simulink model "Controller_without_ref"  (R2015b)
settings: Solver=FixedStepDiscrete  SolverMode=SingleTasking  StartTime=0.0  StopTime=inf  RelTol=1e-3
undefined symbols (not defined in the file or in its folder): Controls, DiscIntNeverNeededParam, GroupMix
libraries: robotlib x34, simulink x6
settings Model: Creator=rasrack  LastModifiedBy=rasrack
settings OptimizationCC: DefaultParameterBehavior=Inlined  UseFloatMulNetSlope=on  InlineInvariantSignals=on  PassReuseOutputArgsAs=Individual arguments  ZeroExternalMemoryAtStartup=off  ZeroInternalMemoryAtStartup=off  NoFixptDivByZeroProtection=on  EfficientFloat2IntCast=on  OptimizeModelRefInitCode=on  LifeSpan=1  MaxStackSize=64
settings HardwareCC: ProdBitPerPointer=32  ProdLargestAtomicFloat=None  ProdIntDivRoundTo=Undefined  ProdEndianess=Unspecified  ProdWordSize=32  ProdHWDeviceType=Generic->Unspecified (assume 32-bit Generic)
settings ModelReferenceCC: EnableParallelModelReferenceBuilds=on
settings RTWCC: SystemTargetFile=ert.tlc  GenCodeOnly=on  TemplateMakefile=ert_default_tmf  Description=Embedded Coder  GenerateReport=on  Toolchain=Catkin  IncludeHyperlinkInReport=on  LaunchReport=on  TargetLang=C++  GenerateTraceInfo=on  GenerateTraceReport=on  GenerateTraceReportSl=on  GenerateTraceReportSf=on  GenerateTraceReportEml=on
settings CodeAppCC: ForceParamTrailComments=on  IgnoreCustomStorageClasses=off  SimulinkDataObjDesc=on  InsertBlockDesc=on  InternalIdentifier=Classic  ReqsInCode=on
settings ERTTargetCC: IncludeMdlTerminateFcn=off  CombineSignalStateStructs=on  MultiInstanceERTCode=on  CodeInterfacePackaging=C++ class  SupportNonFinite=off  SupportVariableSizeSignals=on  InlinedParameterPlacement=NonHierarchical  RootIOFormat=Structure reference  ERTFilePackagingFormat=CompactWithDataFile

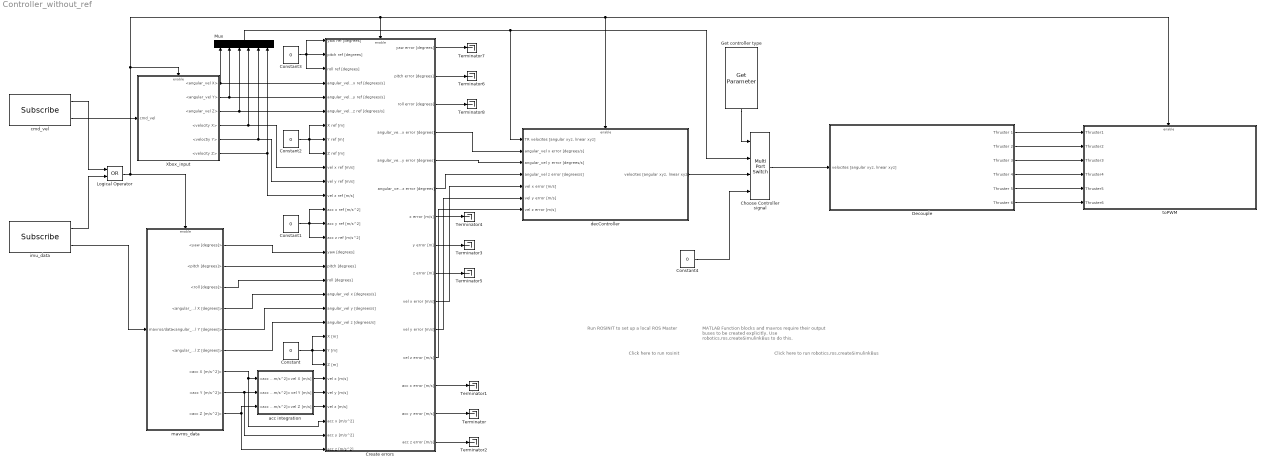
== system Controller_without_ref ==
  note: Click here to run
      | robotics.ros.createSimulinkBus
  note: Run ROSINIT to set up a local ROS Master
  note: MATLAB Function blocks and mavros require their output buses to be created explicitly. Use robotics.ros.createSimulinkBus to do this.
  note: Click here to run
      | rosinit
  Choose Controller signal : MultiPortSwitch  DataPortOrder=Specify indices  DataPortIndices={0,1,2}
  Constant{,1..4} (5 alike) : Constant  Value=0
  Create errors : Subsystem
  Decouple : Subsystem
  Get controller type : robotlib/Get Parameter  SourceLibraryInfo=This block requires Robotics System Toolbox  ParameterSource=Select from ROS network  ParameterName=/matlab_controller/controller  ParameterType=int32  ParameterInitialValue=0  SampleTime=-1  ShowErrorCodeOutput=off  ModelName=Controller_without_ref  BlockId=ParamGet_Controller_without_ref_106
  Logical Operator : Logic  Operator=OR  AllPortsSameDT=off  OutDataTypeStr=boolean
  Mux : Mux  Inputs=6
  Terminator{,1..8} (9 alike) : Terminator
  Xbox_input : Subsystem
  acc integration : Subsystem
  cmd_vel : robotlib/Subscribe  SourceLibraryInfo=This block requires Robotics System Toolbox  topicSource=Select from ROS network  topic=/cmd_vel  messageType=geometry_msgs/Twist  sampleTime=-1  messageQueueLength=10
  decController : Subsystem
  imu_data : robotlib/Subscribe  SourceLibraryInfo=This block requires Robotics System Toolbox  topicSource=Select from ROS network  topic=/mavros/imu/data  messageType=sensor_msgs/Imu  sampleTime=-1  messageQueueLength=10
  mavros_data : Subsystem  TreatAsAtomicUnit=on
  toPWM : Subsystem
  wires:
  cmd_vel/2 -> Xbox_input/1(cmd_vel)
  cmd_vel/1 -> Logical Operator/1
  imu_data/1 -> Logical Operator/2
  imu_data/2 -> mavros_data/1(mavros/data)
  Get controller type/1 -> Choose Controller signal/1
  Xbox_input/1(<angular_vel X>) -> Create errors/4(angular_vel x ref [degrees/s]), Mux/1
  Xbox_input/2(<angular_vel Y>) -> Mux/2, Create errors/5(angular_vel y ref [degrees/s])
  Xbox_input/3("<angular_vel Z> ") -> Mux/3, Create errors/6("angular_vel z ref [degrees/s] ")
  Xbox_input/4(<velocity X>) -> Mux/4, Create errors/10(vel x ref [m/s])
  Xbox_input/5(<veloctiy Y>) -> Mux/5, Create errors/11(vel y ref [m/s])
  Xbox_input/6(<velocity Z>) -> Create errors/12(vel z ref [m/s]), Mux/6
  mavros_data/1(<yaw [degrees]>) -> Create errors/16("yaw [degrees]  ")
  mavros_data/2(<pitch [degrees]>) -> Create errors/17(pitch [degrees])
  mavros_data/3(<roll [degrees]>) -> Create errors/18(roll [degrees])
  mavros_data/4(<angular_vel X [degrees]>) -> Create errors/19("angular_vel x [degrees/s]  ")
  mavros_data/5(<angular_vel Y [degrees]>) -> Create errors/20("angular_vel y [degrees/s] ")
  mavros_data/6(<angular_vel Z [degrees]>) -> Create errors/21(angular_vel z [degrees/s])
  Constant/1 -> Create errors/22(X [m]), Create errors/24(Z [m]), Create errors/23(Y [m])
  acc integration/2(vel Y [m/s]) -> Create errors/26(vel y [m/s])
  acc integration/1("vel X [m/s] ") -> Create errors/25(vel x [m/s])
  acc integration/3(vel Z [m/s]) -> Create errors/27(vel z [m/s])
  mavros_data/7(<acc X [m/s^2]>) -> Create errors/28(acc x [m/s^2]), acc integration/1("<acc X [m/s^2]> ")
  mavros_data/8(<acc Y [m/s^2]>) -> Create errors/29(acc y [m/s^2]), acc integration/2(<acc Y [m/s^2]>)
  mavros_data/9(<acc Z [m/s^2]>) -> Create errors/30(acc z [m/s^2]), acc integration/3(<acc Z [m/s^2]>)
  Constant1/1 -> Create errors/15(acc z ref [m/s^2]), Create errors/13(acc x ref [m/s^2]), Create errors/14(acc y ref [m/s^2])
  Constant2/1 -> Create errors/9(Z ref [m]), Create errors/7(X ref [m]), Create errors/8(Y ref [m])
  Constant3/1 -> Create errors/1("yaw ref [degrees] "), Create errors/3(roll ref [degrees]), Create errors/2("pitch ref [degrees] ")
  Mux/1 -> decController/1("TR velocites [angular xyz, linear xyz]  "), Choose Controller signal/2
  Create errors/14(acc y error [m/s]) -> Terminator/1
  Create errors/13(acc x error [m/s]) -> Terminator1/1
  Create errors/15(acc z error [m/s]) -> Terminator2/1
  Create errors/8(y error [m]) -> Terminator3/1
  Create errors/7(x error [m/s]) -> Terminator4/1
  Create errors/9(z error [m]) -> Terminator5/1
  Create errors/2(pitch error [degrees]) -> Terminator6/1
  Create errors/1(yaw error [degrees]) -> Terminator7/1
  Create errors/3(roll error [degrees]) -> Terminator8/1
  Constant4/1 -> Choose Controller signal/4
  Choose Controller signal/1 -> Decouple/1("velocites [angular xyz, linear xyz]    ")
  Create errors/4(angular_vel x error [degrees]) -> decController/2("angular_vel x error [degrees/s] ")
  Create errors/5(angular_vel y error [degrees]) -> decController/3(angular_vel y error [degrees/s])
  Create errors/6(angular_vel z error [degrees]) -> decController/4(angular_vel z error [degrees/s])
  Create errors/10(vel x error [m/s]) -> decController/5("vel x error [m/s] ")
  Create errors/11(vel y error [m/s]) -> decController/6("vel y error [m/s] ")
  Create errors/12(vel z error [m/s]) -> decController/7("vel z error [m/s] ")
  decController/1("velocites [angular xyz, linear xyz]") -> Choose Controller signal/3
  Logical Operator/1 -> mavros_data/Enable, Create errors/Enable, toPWM/Enable, decController/Enable, Xbox_input/Enable
  Decouple/3(Thruster 3) -> toPWM/3(Thruster3)
  Decouple/2(Thruster 2) -> toPWM/2(Thruster2)
  Decouple/5(Thruster 5) -> toPWM/5(Thruster5)
  Decouple/1(Thruster 1) -> toPWM/1(Thruster1)
  Decouple/4(Thruster 4) -> toPWM/4(Thruster4)
  Decouple/6(Thruster 6) -> toPWM/6(Thruster6)

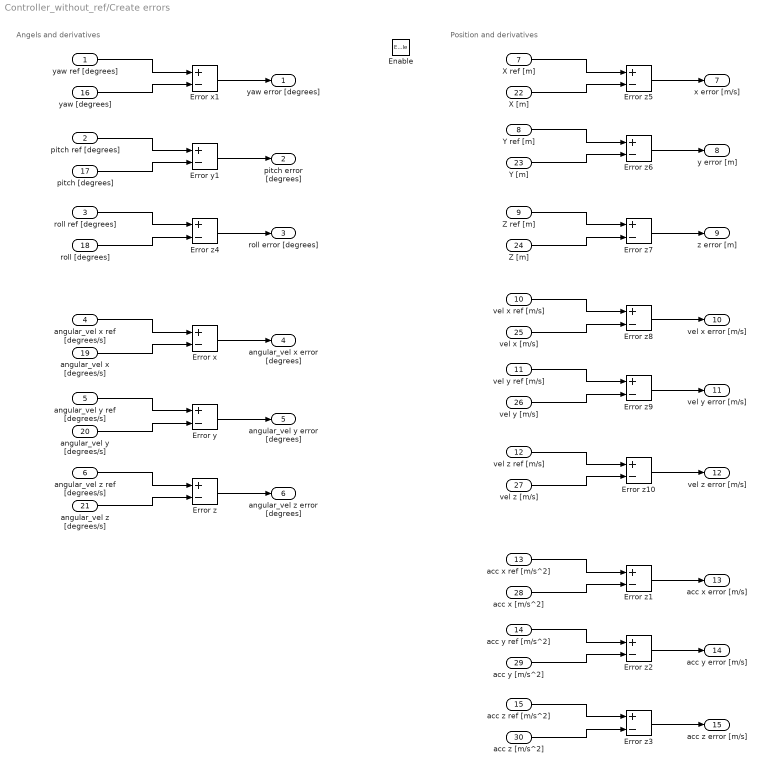
== system Controller_without_ref/Create errors ==
  note: Position and derivatives
  note: Angels and derivatives
  "yaw ref [degrees] " : Inport
  "pitch ref [degrees] " : Inport  Port=2
  roll ref [degrees] : Inport  Port=3
  angular_vel x ref [degrees/s] : Inport  Port=4
  angular_vel y ref [degrees/s] : Inport  Port=5
  "angular_vel z ref [degrees/s] " : Inport  Port=6
  X ref [m] : Inport  Port=7
  Y ref [m] : Inport  Port=8
  Z ref [m] : Inport  Port=9
  vel x ref [m/s] : Inport  Port=10
  vel y ref [m/s] : Inport  Port=11
  vel z ref [m/s] : Inport  Port=12
  acc x ref [m/s^2] : Inport  Port=13
  acc y ref [m/s^2] : Inport  Port=14
  acc z ref [m/s^2] : Inport  Port=15
  "yaw [degrees]  " : Inport  Port=16
  pitch [degrees] : Inport  Port=17
  roll [degrees] : Inport  Port=18
  "angular_vel x [degrees/s]  " : Inport  Port=19
  "angular_vel y [degrees/s] " : Inport  Port=20
  angular_vel z [degrees/s] : Inport  Port=21
  X [m] : Inport  Port=22
  Y [m] : Inport  Port=23
  Z [m] : Inport  Port=24
  vel x [m/s] : Inport  Port=25
  vel y [m/s] : Inport  Port=26
  vel z [m/s] : Inport  Port=27
  acc x [m/s^2] : Inport  Port=28
  acc y [m/s^2] : Inport  Port=29
  acc z [m/s^2] : Inport  Port=30
  Enable : EnablePort
  Error x : Sum  Inputs=+-
  Error x1 : Sum  Inputs=+-
  Error y : Sum  Inputs=+-
  Error y1 : Sum  Inputs=+-
  Error z{,1..10} (11 alike) : Sum  Inputs=+-
  yaw error [degrees] : Outport
  pitch error [degrees] : Outport  Port=2
  roll error [degrees] : Outport  Port=3
  angular_vel x error [degrees] : Outport  Port=4
  angular_vel y error [degrees] : Outport  Port=5
  angular_vel z error [degrees] : Outport  Port=6
  x error [m/s] : Outport  Port=7
  y error [m] : Outport  Port=8
  z error [m] : Outport  Port=9
  vel x error [m/s] : Outport  Port=10
  vel y error [m/s] : Outport  Port=11
  vel z error [m/s] : Outport  Port=12
  acc x error [m/s] : Outport  Port=13
  acc y error [m/s] : Outport  Port=14
  acc z error [m/s] : Outport  Port=15
  wires:
  angular_vel x ref [degrees/s]/1 -> Error x/1
  "angular_vel x [degrees/s]  "/1 -> Error x/2
  Error x/1 -> angular_vel x error [degrees]/1
  angular_vel y ref [degrees/s]/1 -> Error y/1
  "angular_vel y [degrees/s] "/1 -> Error y/2
  Error y/1 -> angular_vel y error [degrees]/1
  "angular_vel z ref [degrees/s] "/1 -> Error z/1
  angular_vel z [degrees/s]/1 -> Error z/2
  Error z/1 -> angular_vel z error [degrees]/1
  acc x ref [m/s^2]/1 -> Error z1/1
  acc x [m/s^2]/1 -> Error z1/2
  Error z1/1 -> acc x error [m/s]/1
  acc y ref [m/s^2]/1 -> Error z2/1
  acc y [m/s^2]/1 -> Error z2/2
  Error z2/1 -> acc y error [m/s]/1
  acc z ref [m/s^2]/1 -> Error z3/1
  acc z [m/s^2]/1 -> Error z3/2
  Error z3/1 -> acc z error [m/s]/1
  "yaw ref [degrees] "/1 -> Error x1/1
  "yaw [degrees]  "/1 -> Error x1/2
  Error x1/1 -> yaw error [degrees]/1
  "pitch ref [degrees] "/1 -> Error y1/1
  pitch [degrees]/1 -> Error y1/2
  Error y1/1 -> pitch error [degrees]/1
  roll ref [degrees]/1 -> Error z4/1
  roll [degrees]/1 -> Error z4/2
  Error z4/1 -> roll error [degrees]/1
  X ref [m]/1 -> Error z5/1
  X [m]/1 -> Error z5/2
  Error z5/1 -> x error [m/s]/1
  Y ref [m]/1 -> Error z6/1
  Y [m]/1 -> Error z6/2
  Error z6/1 -> y error [m]/1
  Z ref [m]/1 -> Error z7/1
  Z [m]/1 -> Error z7/2
  Error z7/1 -> z error [m]/1
  vel x ref [m/s]/1 -> Error z8/1
  vel x [m/s]/1 -> Error z8/2
  Error z8/1 -> vel x error [m/s]/1
  vel y ref [m/s]/1 -> Error z9/1
  vel y [m/s]/1 -> Error z9/2
  Error z9/1 -> vel y error [m/s]/1
  vel z ref [m/s]/1 -> Error z10/1
  vel z [m/s]/1 -> Error z10/2
  Error z10/1 -> vel z error [m/s]/1

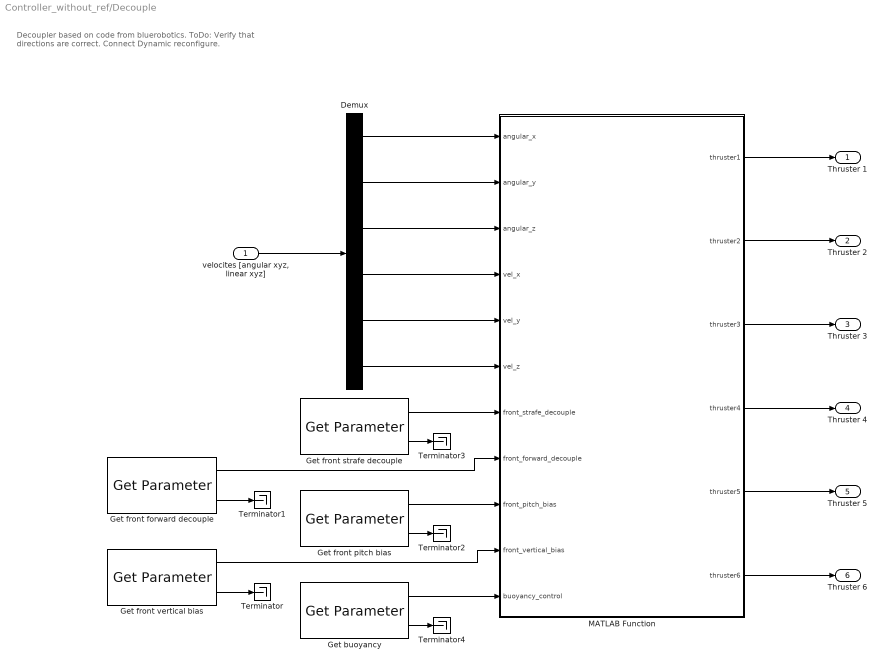
== system Controller_without_ref/Decouple ==
  note: Decoupler based on code from bluerobotics.
      | ToDo:
      | Verify that directions are correct.
      | Connect Dynamic reconfigure.
  "velocites [angular xyz, linear xyz]    " : Inport
  Demux : Demux  Outputs=6
  Get buoyancy : robotlib/Get Parameter  SourceLibraryInfo=This block requires Robotics System Toolbox  ParameterSource=Select from ROS network  ParameterName=/matlab_controller/buoyancy_control  ParameterType=double  ParameterInitialValue=0.0  SampleTime=-1  ShowErrorCodeOutput=on  ModelName=Controller_without_ref  BlockId=ParamGet_Controller_without_ref_462
  Get front forward decouple : robotlib/Get Parameter  SourceLibraryInfo=This block requires Robotics System Toolbox  ParameterSource=Select from ROS network  ParameterName=/matlab_controller/front_forward_decouple  ParameterType=double  ParameterInitialValue=0.0  SampleTime=-1  ShowErrorCodeOutput=on  ModelName=Controller_without_ref  BlockId=ParamGet_Controller_without_ref_463
  Get front pitch bias : robotlib/Get Parameter  SourceLibraryInfo=This block requires Robotics System Toolbox  ParameterSource=Select from ROS network  ParameterName=/matlab_controller/front_pitch_bias  ParameterType=double  ParameterInitialValue=0.0  SampleTime=-1  ShowErrorCodeOutput=on  ModelName=Controller_without_ref  BlockId=ParamGet_Controller_without_ref_464
  Get front strafe decouple : robotlib/Get Parameter  SourceLibraryInfo=This block requires Robotics System Toolbox  ParameterSource=Select from ROS network  ParameterName=/matlab_controller/front_strafe_decouple  ParameterType=double  ParameterInitialValue=0.0  SampleTime=-1  ShowErrorCodeOutput=on  ModelName=Controller_without_ref  BlockId=ParamGet_Controller_without_ref_465
  Get front vertical bias : robotlib/Get Parameter  SourceLibraryInfo=This block requires Robotics System Toolbox  ParameterSource=Select from ROS network  ParameterName=/matlab_controller/front_vertical_bias  ParameterType=double  ParameterInitialValue=0.0  SampleTime=-1  ShowErrorCodeOutput=on  ModelName=Controller_without_ref  BlockId=ParamGet_Controller_without_ref_466
  MATLAB Function : MATLAB Function  TreatAsAtomicUnit=on
  Terminator{,1..4} (5 alike) : Terminator
  Thruster 1 : Outport
  Thruster 2 : Outport  Port=2
  Thruster 3 : Outport  Port=3
  Thruster 4 : Outport  Port=4
  Thruster 5 : Outport  Port=5
  Thruster 6 : Outport  Port=6
  wires:
  MATLAB Function/1(thruster1) -> Thruster 1/1
  Get buoyancy/1 -> MATLAB Function/11(buoyancy_control)
  Get front vertical bias/1 -> MATLAB Function/10(front_vertical_bias)
  Get front pitch bias/1 -> MATLAB Function/9(front_pitch_bias)
  Get front forward decouple/1 -> MATLAB Function/8(front_forward_decouple)
  Get front strafe decouple/1 -> MATLAB Function/7(front_strafe_decouple)
  Demux/5 -> MATLAB Function/5(vel_y)
  Demux/6 -> MATLAB Function/6(vel_z)
  Demux/4 -> MATLAB Function/4(vel_x)
  Demux/3 -> MATLAB Function/3(angular_z)
  Demux/2 -> MATLAB Function/2(angular_y)
  Demux/1 -> MATLAB Function/1(angular_x)
  MATLAB Function/6(thruster6) -> Thruster 6/1
  MATLAB Function/5(thruster5) -> Thruster 5/1
  MATLAB Function/4(thruster4) -> Thruster 4/1
  MATLAB Function/3(thruster3) -> Thruster 3/1
  MATLAB Function/2(thruster2) -> Thruster 2/1
  Get front vertical bias/2 -> Terminator/1
  Get front forward decouple/2 -> Terminator1/1
  Get front pitch bias/2 -> Terminator2/1
  Get front strafe decouple/2 -> Terminator3/1
  Get buoyancy/2 -> Terminator4/1
  "velocites [angular xyz, linear xyz]    "/1 -> Demux/1

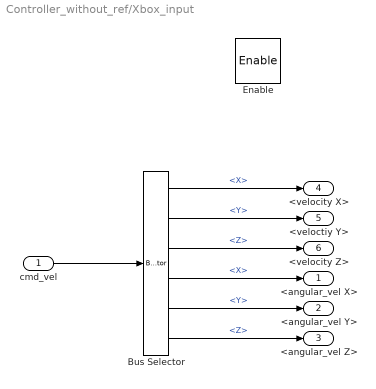
== system Controller_without_ref/Xbox_input ==
  cmd_vel : Inport
  Enable : EnablePort
  Bus Selector : BusSelector  OutputSignals=Linear.X,Linear.Y,Linear.Z,Angular.X,Angular.Y,Angular.Z
  <angular_vel X> : Outport
  <angular_vel Y> : Outport  Port=2
  "<angular_vel Z> " : Outport  Port=3
  <velocity X> : Outport  Port=4
  <veloctiy Y> : Outport  Port=5
  <velocity Z> : Outport  Port=6
  wires:
  cmd_vel/1 -> Bus Selector/1
  Bus Selector/2 -> <veloctiy Y>/1  "<Y>"
  Bus Selector/1 -> <velocity X>/1  "<X>"
  Bus Selector/5 -> <angular_vel Y>/1  "<Y>"
  Bus Selector/3 -> <velocity Z>/1  "<Z>"
  Bus Selector/6 -> "<angular_vel Z> "/1  "<Z>"
  Bus Selector/4 -> <angular_vel X>/1  "<X>"

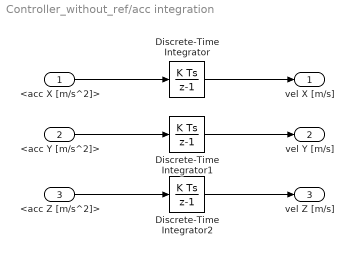
== system Controller_without_ref/acc integration ==
  "<acc X [m/s^2]> " : Inport
  <acc Y [m/s^2]> : Inport  Port=2
  <acc Z [m/s^2]> : Inport  Port=3
  Discrete-Time Integrator : DiscreteIntegrator  InitialConditionSetting=State (most efficient)  SampleTime=-1  ICPrevOutput=DiscIntNeverNeededParam  ICPrevScaledInput=DiscIntNeverNeededParam
  Discrete-Time Integrator1 : DiscreteIntegrator  InitialConditionSetting=State (most efficient)  SampleTime=-1  ICPrevOutput=DiscIntNeverNeededParam  ICPrevScaledInput=DiscIntNeverNeededParam
  Discrete-Time Integrator2 : DiscreteIntegrator  InitialConditionSetting=State (most efficient)  SampleTime=-1  ICPrevOutput=DiscIntNeverNeededParam  ICPrevScaledInput=DiscIntNeverNeededParam
  "vel X [m/s] " : Outport
  vel Y [m/s] : Outport  Port=2
  vel Z [m/s] : Outport  Port=3
  wires:
  "<acc X [m/s^2]> "/1 -> Discrete-Time Integrator/1
  <acc Y [m/s^2]>/1 -> Discrete-Time Integrator1/1
  <acc Z [m/s^2]>/1 -> Discrete-Time Integrator2/1
  Discrete-Time Integrator/1 -> "vel X [m/s] "/1
  Discrete-Time Integrator1/1 -> vel Y [m/s]/1
  Discrete-Time Integrator2/1 -> vel Z [m/s]/1

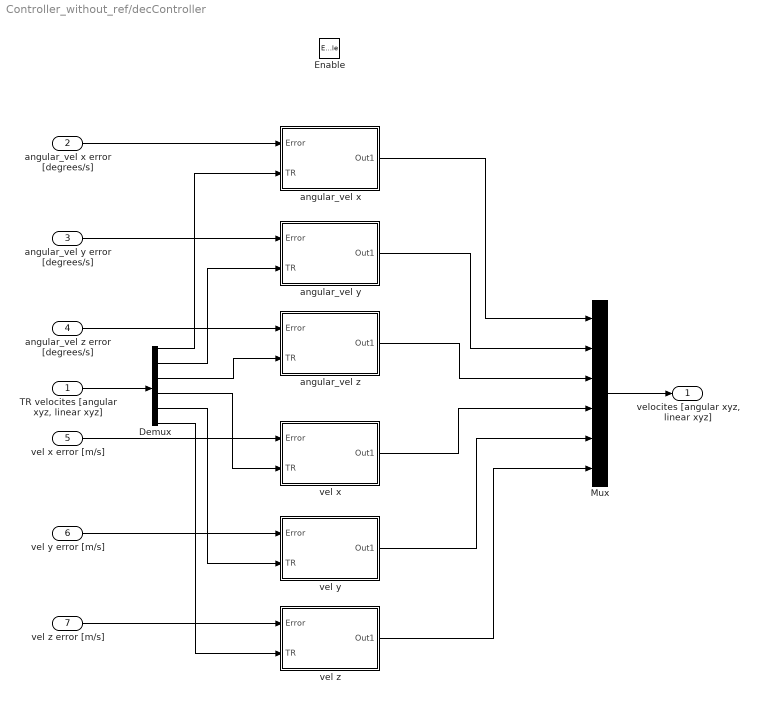
== system Controller_without_ref/decController ==
  "TR velocites [angular xyz, linear xyz]  " : Inport
  "angular_vel x error [degrees/s] " : Inport  Port=2
  angular_vel y error [degrees/s] : Inport  Port=3
  angular_vel z error [degrees/s] : Inport  Port=4
  "vel x error [m/s] " : Inport  Port=5
  "vel y error [m/s] " : Inport  Port=6
  "vel z error [m/s] " : Inport  Port=7
  Enable : EnablePort  OutDataTypeStr=boolean
  Demux : Demux  Outputs=6
  Mux : Mux  Inputs=6
  angular_vel x : Subsystem
  angular_vel y : Subsystem
  angular_vel z : Subsystem
  vel x : Subsystem
  vel y : Subsystem
  vel z : Subsystem
  "velocites [angular xyz, linear xyz]" : Outport
  wires:
  "angular_vel x error [degrees/s] "/1 -> angular_vel x/1(Error)
  angular_vel y error [degrees/s]/1 -> angular_vel y/1(Error)
  angular_vel z error [degrees/s]/1 -> angular_vel z/1(Error)
  "vel x error [m/s] "/1 -> vel x/1(Error)
  "vel y error [m/s] "/1 -> vel y/1(Error)
  "vel z error [m/s] "/1 -> vel z/1(Error)
  vel z/1(Out1) -> Mux/6
  angular_vel x/1(Out1) -> Mux/1
  angular_vel y/1(Out1) -> Mux/2
  angular_vel z/1(Out1) -> Mux/3
  vel x/1(Out1) -> Mux/4
  vel y/1(Out1) -> Mux/5
  Mux/1 -> "velocites [angular xyz, linear xyz]"/1
  "TR velocites [angular xyz, linear xyz]  "/1 -> Demux/1
  Demux/1 -> angular_vel x/2(TR)
  Demux/2 -> angular_vel y/2(TR)
  Demux/3 -> angular_vel z/2(TR)
  Demux/4 -> vel x/2(TR)
  Demux/5 -> vel y/2(TR)
  Demux/6 -> vel z/2(TR)

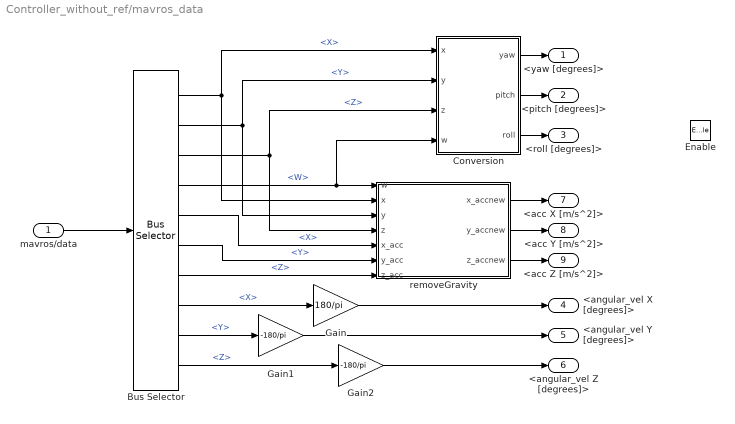
== system Controller_without_ref/mavros_data ==
  mavros/data : Inport
  Enable : EnablePort
  Bus Selector : BusSelector  OutputSignals=Orientation.X,Orientation.Y,Orientation.Z,Orientation.W,LinearAcceleration.X,LinearAcceleration.Y,LinearAcceleration.Z,AngularVelocity.X,AngularVelocity.Y,AngularVelocity.Z
  Conversion : MATLAB Function  TreatAsAtomicUnit=on
  Gain : Gain  Gain=180/pi
  Gain1 : Gain  Gain=-180/pi
  Gain2 : Gain  Gain=-180/pi
  removeGravity : MATLAB Function  TreatAsAtomicUnit=on
  <yaw [degrees]> : Outport
  <pitch [degrees]> : Outport  Port=2
  <roll [degrees]> : Outport  Port=3
  <angular_vel X [degrees]> : Outport  Port=4
  <angular_vel Y [degrees]> : Outport  Port=5
  <angular_vel Z [degrees]> : Outport  Port=6
  <acc X [m/s^2]> : Outport  Port=7
  <acc Y [m/s^2]> : Outport  Port=8
  <acc Z [m/s^2]> : Outport  Port=9
  wires:
  mavros/data/1 -> Bus Selector/1
  Bus Selector/1 -> removeGravity/2(x), Conversion/1(x)  "<X>"
  Bus Selector/2 -> removeGravity/3(y), Conversion/2(y)  "<Y>"
  Bus Selector/3 -> removeGravity/4(z), Conversion/3(z)  "<Z>"
  Bus Selector/4 -> removeGravity/1(w), Conversion/4(w)  "<W>"
  Conversion/1(yaw) -> <yaw [degrees]>/1
  Conversion/3(roll) -> <roll [degrees]>/1
  Conversion/2(pitch) -> <pitch [degrees]>/1
  Bus Selector/8 -> Gain/1  "<X>"
  Bus Selector/9 -> Gain1/1  "<Y>"
  Bus Selector/10 -> Gain2/1  "<Z>"
  Bus Selector/5 -> removeGravity/5(x_acc)  "<X>"
  Bus Selector/6 -> removeGravity/6(y_acc)  "<Y>"
  Bus Selector/7 -> removeGravity/7(z_acc)  "<Z>"
  removeGravity/3(z_accnew) -> <acc Z [m/s^2]>/1
  removeGravity/2(y_accnew) -> <acc Y [m/s^2]>/1
  removeGravity/1(x_accnew) -> <acc X [m/s^2]>/1
  Gain/1 -> <angular_vel X [degrees]>/1
  Gain1/1 -> <angular_vel Y [degrees]>/1
  Gain2/1 -> <angular_vel Z [degrees]>/1

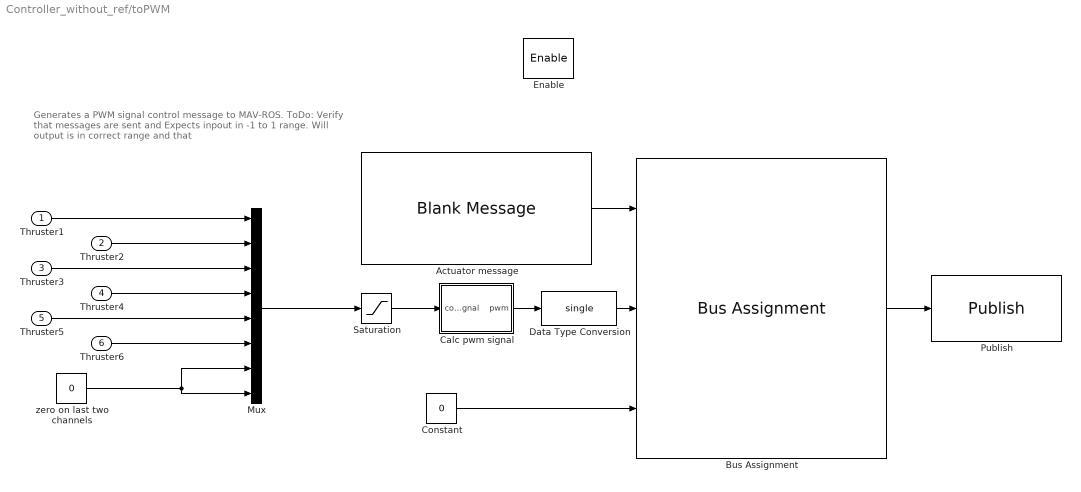
== system Controller_without_ref/toPWM ==
  note: Generates a PWM signal control message to
      | MAV-ROS.
      | ToDo:
      | Verify that messages are sent and
      | Expects inpout in -1 to 1 range.
      | Will output is in correct range and that
  Thruster1 : Inport  PortDimensions=1
  Thruster2 : Inport  Port=2  OutDataTypeStr=double  PortDimensions=1
  Thruster3 : Inport  Port=3  PortDimensions=1
  Thruster4 : Inport  Port=4  PortDimensions=1
  Thruster5 : Inport  Port=5  PortDimensions=1
  Thruster6 : Inport  Port=6  PortDimensions=1
  Enable : EnablePort  OutDataTypeStr=boolean
  "Actuator message " : robotlib/Blank Message  SourceLibraryInfo=This block requires Robotics System Toolbox  messageType=mavros_msgs/ActuatorControl  SampleTime=inf
  Bus Assignment : BusAssignment  AssignedSignals=Controls,GroupMix
  Calc pwm signal : MATLAB Function  TreatAsAtomicUnit=on
  Constant : Constant  Value=0  OutDataTypeStr=uint8
  Data Type Conversion : DataTypeConversion  OutDataTypeStr=single
  Mux : Mux  Inputs=8
  Publish : robotlib/Publish  SourceLibraryInfo=This block requires Robotics System Toolbox  topicSource=Select from ROS network  topic=/mavros/actuator_control  messageType=mavros_msgs/ActuatorControl  messageQueueLength=1
  Saturation : Saturate  UpperLimit=1  LowerLimit=-1
  zero on last two channels : Constant  Value=0  OutDataTypeStr=double
  wires:
  "Actuator message "/1 -> Bus Assignment/1
  Constant/1 -> Bus Assignment/3
  Bus Assignment/1 -> Publish/1
  Saturation/1 -> Calc pwm signal/1(controlsignal)
  Thruster1/1 -> Mux/1
  Mux/1 -> Saturation/1
  zero on last two channels/1 -> Mux/7, Mux/8
  Thruster4/1 -> Mux/4
  Thruster6/1 -> Mux/6
  Thruster5/1 -> Mux/5
  Thruster2/1 -> Mux/2
  Thruster3/1 -> Mux/3
  Data Type Conversion/1 -> Bus Assignment/2
  Calc pwm signal/1(pwm) -> Data Type Conversion/1

== system Controller_without_ref/decController/angular_vel x ==
  Error : Inport
  TR : Inport  Port=2
  PID Controller : simulink/Continuous/PID Controller  Controller=PID  TimeDomain=Discrete-time  SampleTime=-1  IntegratorMethod=Forward Euler  FilterMethod=Forward Euler  Form=Parallel  UseFilter=on  ControllerParametersSource=external  P=1  I=1  D=0  N=100  InitialConditionSource=internal  InitialConditionForIntegrator=0  InitialConditionForFilter=0  ExternalReset=none  LimitOutput=on  UpperSaturationLimit=1  LowerSaturationLimit=-1  LinearizeAsGain=on  AntiWindupMode=clamping  Kb=1  TrackingMode=on  Kt=1  SaturateOnIntegerOverflow=on  PParamMin=[]  PParamMax=[]  IParamMin=[]  IParamMax=[]  DParamMin=[]  DParamMax=[]  NParamMin=[]  NParamMax=[]  KbParamMin=[]  KbParamMax=[]  KtParamMin=[]  KtParamMax=[]  POutMin=[]  POutMax=[]  IOutMin=[]  IOutMax=[]  DOutMin=[]  DOutMax=[]  NOutMin=[]  NOutMax=[]  KbOutMin=[]  KbOutMax=[]  KtOutMin=[]  KtOutMax=[]  IntegratorOutMin=[]  IntegratorOutMax=[]  FilterOutMin=[]  FilterOutMax=[]  SumOutMin=[]  SumOutMax=[]  SumI1OutMin=[]  SumI1OutMax=[]  SumI2OutMin=[]  SumI2OutMax=[]  SumI3OutMin=[]  SumI3OutMax=[]  SumDOutMin=[]  SumDOutMax=[]  SaturationOutMin=[]  SaturationOutMax=[]  SaturationOutDataTypeStr=double  IntegratorContinuousStateAttributes=''  IntegratorStateMustResolveToSignalObject=off  IntegratorRTWStateStorageClass=Auto  FilterContinuousStateAttributes=''  FilterStateMustResolveToSignalObject=off  FilterRTWStateStorageClass=Auto  DifferentiatorICPrevScaledInput=0  DifferentiatorOutMin=[]  DifferentiatorOutMax=[]
  Retrive PID-Parameters : Subsystem
  Out1 : Outport
  wires:
  Retrive PID-Parameters/3(D) -> PID Controller/4
  Retrive PID-Parameters/2(I) -> PID Controller/3
  Retrive PID-Parameters/4(N) -> PID Controller/5
  Retrive PID-Parameters/1(P) -> PID Controller/2
  TR/1 -> PID Controller/6
  Error/1 -> PID Controller/1
  PID Controller/1 -> Out1/1

== system Controller_without_ref/decController/angular_vel y ==
  Error : Inport
  TR : Inport  Port=2
  PID Controller : simulink/Continuous/PID Controller  Controller=PID  TimeDomain=Discrete-time  SampleTime=-1  IntegratorMethod=Forward Euler  FilterMethod=Forward Euler  Form=Parallel  UseFilter=on  ControllerParametersSource=external  P=1  I=1  D=0  N=100  InitialConditionSource=internal  InitialConditionForIntegrator=0  InitialConditionForFilter=0  ExternalReset=none  LimitOutput=on  UpperSaturationLimit=1  LowerSaturationLimit=-1  LinearizeAsGain=on  AntiWindupMode=clamping  Kb=1  TrackingMode=on  Kt=1  SaturateOnIntegerOverflow=on  PParamMin=[]  PParamMax=[]  IParamMin=[]  IParamMax=[]  DParamMin=[]  DParamMax=[]  NParamMin=[]  NParamMax=[]  KbParamMin=[]  KbParamMax=[]  KtParamMin=[]  KtParamMax=[]  POutMin=[]  POutMax=[]  IOutMin=[]  IOutMax=[]  DOutMin=[]  DOutMax=[]  NOutMin=[]  NOutMax=[]  KbOutMin=[]  KbOutMax=[]  KtOutMin=[]  KtOutMax=[]  IntegratorOutMin=[]  IntegratorOutMax=[]  FilterOutMin=[]  FilterOutMax=[]  SumOutMin=[]  SumOutMax=[]  SumI1OutMin=[]  SumI1OutMax=[]  SumI2OutMin=[]  SumI2OutMax=[]  SumI3OutMin=[]  SumI3OutMax=[]  SumDOutMin=[]  SumDOutMax=[]  SaturationOutMin=[]  SaturationOutMax=[]  IntegratorContinuousStateAttributes=''  IntegratorStateMustResolveToSignalObject=off  IntegratorRTWStateStorageClass=Auto  FilterContinuousStateAttributes=''  FilterStateMustResolveToSignalObject=off  FilterRTWStateStorageClass=Auto  DifferentiatorICPrevScaledInput=0  DifferentiatorOutMin=[]  DifferentiatorOutMax=[]
  Retrive PID-Parameters : Subsystem
  Out1 : Outport
  wires:
  Retrive PID-Parameters/3(D) -> PID Controller/4
  Retrive PID-Parameters/2(I) -> PID Controller/3
  Retrive PID-Parameters/4(N) -> PID Controller/5
  Retrive PID-Parameters/1(P) -> PID Controller/2
  TR/1 -> PID Controller/6
  Error/1 -> PID Controller/1
  PID Controller/1 -> Out1/1

== system Controller_without_ref/decController/angular_vel z ==
  Error : Inport
  TR : Inport  Port=2
  PID Controller : simulink/Continuous/PID Controller  Controller=PID  TimeDomain=Discrete-time  SampleTime=-1  IntegratorMethod=Forward Euler  FilterMethod=Forward Euler  Form=Parallel  UseFilter=on  ControllerParametersSource=external  P=1  I=1  D=0  N=100  InitialConditionSource=internal  InitialConditionForIntegrator=0  InitialConditionForFilter=0  ExternalReset=none  LimitOutput=on  UpperSaturationLimit=1  LowerSaturationLimit=-1  LinearizeAsGain=on  AntiWindupMode=clamping  Kb=1  TrackingMode=on  Kt=1  SaturateOnIntegerOverflow=on  PParamMin=[]  PParamMax=[]  IParamMin=[]  IParamMax=[]  DParamMin=[]  DParamMax=[]  NParamMin=[]  NParamMax=[]  KbParamMin=[]  KbParamMax=[]  KtParamMin=[]  KtParamMax=[]  POutMin=[]  POutMax=[]  IOutMin=[]  IOutMax=[]  DOutMin=[]  DOutMax=[]  NOutMin=[]  NOutMax=[]  KbOutMin=[]  KbOutMax=[]  KtOutMin=[]  KtOutMax=[]  IntegratorOutMin=[]  IntegratorOutMax=[]  FilterOutMin=[]  FilterOutMax=[]  SumOutMin=[]  SumOutMax=[]  SumI1OutMin=[]  SumI1OutMax=[]  SumI2OutMin=[]  SumI2OutMax=[]  SumI3OutMin=[]  SumI3OutMax=[]  SumDOutMin=[]  SumDOutMax=[]  SaturationOutMin=[]  SaturationOutMax=[]  IntegratorContinuousStateAttributes=''  IntegratorStateMustResolveToSignalObject=off  IntegratorRTWStateStorageClass=Auto  FilterContinuousStateAttributes=''  FilterStateMustResolveToSignalObject=off  FilterRTWStateStorageClass=Auto  DifferentiatorICPrevScaledInput=0  DifferentiatorOutMin=[]  DifferentiatorOutMax=[]
  Retrive PID-Parameters : Subsystem
  Out1 : Outport
  wires:
  Retrive PID-Parameters/3(D) -> PID Controller/4
  Retrive PID-Parameters/2(I) -> PID Controller/3
  Retrive PID-Parameters/4(N) -> PID Controller/5
  Retrive PID-Parameters/1(P) -> PID Controller/2
  TR/1 -> PID Controller/6
  Error/1 -> PID Controller/1
  PID Controller/1 -> Out1/1

== system Controller_without_ref/decController/vel x ==
  Error : Inport
  TR : Inport  Port=2
  PID Controller : simulink/Continuous/PID Controller  Controller=PID  TimeDomain=Discrete-time  SampleTime=-1  IntegratorMethod=Forward Euler  FilterMethod=Forward Euler  Form=Parallel  UseFilter=on  ControllerParametersSource=external  P=1  I=1  D=0  N=100  InitialConditionSource=internal  InitialConditionForIntegrator=0  InitialConditionForFilter=0  ExternalReset=none  LimitOutput=on  UpperSaturationLimit=1  LowerSaturationLimit=-1  LinearizeAsGain=on  AntiWindupMode=clamping  Kb=1  TrackingMode=on  Kt=1  SaturateOnIntegerOverflow=on  PParamMin=[]  PParamMax=[]  IParamMin=[]  IParamMax=[]  DParamMin=[]  DParamMax=[]  NParamMin=[]  NParamMax=[]  KbParamMin=[]  KbParamMax=[]  KtParamMin=[]  KtParamMax=[]  POutMin=[]  POutMax=[]  IOutMin=[]  IOutMax=[]  DOutMin=[]  DOutMax=[]  NOutMin=[]  NOutMax=[]  KbOutMin=[]  KbOutMax=[]  KtOutMin=[]  KtOutMax=[]  IntegratorOutMin=[]  IntegratorOutMax=[]  FilterOutMin=[]  FilterOutMax=[]  SumOutMin=[]  SumOutMax=[]  SumI1OutMin=[]  SumI1OutMax=[]  SumI2OutMin=[]  SumI2OutMax=[]  SumI3OutMin=[]  SumI3OutMax=[]  SumDOutMin=[]  SumDOutMax=[]  SaturationOutMin=[]  SaturationOutMax=[]  IntegratorContinuousStateAttributes=''  IntegratorStateMustResolveToSignalObject=off  IntegratorRTWStateStorageClass=Auto  FilterContinuousStateAttributes=''  FilterStateMustResolveToSignalObject=off  FilterRTWStateStorageClass=Auto  DifferentiatorICPrevScaledInput=0  DifferentiatorOutMin=[]  DifferentiatorOutMax=[]
  Retrive PID-Parameters : Subsystem
  Out1 : Outport
  wires:
  Retrive PID-Parameters/3(D) -> PID Controller/4
  Retrive PID-Parameters/2(I) -> PID Controller/3
  Retrive PID-Parameters/4(N) -> PID Controller/5
  Retrive PID-Parameters/1(P) -> PID Controller/2
  TR/1 -> PID Controller/6
  Error/1 -> PID Controller/1
  PID Controller/1 -> Out1/1

== system Controller_without_ref/decController/vel y ==
  Error : Inport
  TR : Inport  Port=2
  PID Controller : simulink/Continuous/PID Controller  Controller=PID  TimeDomain=Discrete-time  SampleTime=-1  IntegratorMethod=Forward Euler  FilterMethod=Forward Euler  Form=Parallel  UseFilter=on  ControllerParametersSource=external  P=1  I=1  D=0  N=100  InitialConditionSource=internal  InitialConditionForIntegrator=0  InitialConditionForFilter=0  ExternalReset=none  LimitOutput=on  UpperSaturationLimit=1  LowerSaturationLimit=-1  LinearizeAsGain=on  AntiWindupMode=clamping  Kb=1  TrackingMode=on  Kt=1  SaturateOnIntegerOverflow=on  PParamMin=[]  PParamMax=[]  IParamMin=[]  IParamMax=[]  DParamMin=[]  DParamMax=[]  NParamMin=[]  NParamMax=[]  KbParamMin=[]  KbParamMax=[]  KtParamMin=[]  KtParamMax=[]  POutMin=[]  POutMax=[]  IOutMin=[]  IOutMax=[]  DOutMin=[]  DOutMax=[]  NOutMin=[]  NOutMax=[]  KbOutMin=[]  KbOutMax=[]  KtOutMin=[]  KtOutMax=[]  IntegratorOutMin=[]  IntegratorOutMax=[]  FilterOutMin=[]  FilterOutMax=[]  SumOutMin=[]  SumOutMax=[]  SumI1OutMin=[]  SumI1OutMax=[]  SumI2OutMin=[]  SumI2OutMax=[]  SumI3OutMin=[]  SumI3OutMax=[]  SumDOutMin=[]  SumDOutMax=[]  SaturationOutMin=[]  SaturationOutMax=[]  IntegratorContinuousStateAttributes=''  IntegratorStateMustResolveToSignalObject=off  IntegratorRTWStateStorageClass=Auto  FilterContinuousStateAttributes=''  FilterStateMustResolveToSignalObject=off  FilterRTWStateStorageClass=Auto  DifferentiatorICPrevScaledInput=0  DifferentiatorOutMin=[]  DifferentiatorOutMax=[]
  Retrive PID-Parameters : Subsystem
  Out1 : Outport
  wires:
  Retrive PID-Parameters/3(D) -> PID Controller/4
  Retrive PID-Parameters/2(I) -> PID Controller/3
  Retrive PID-Parameters/4(N) -> PID Controller/5
  Retrive PID-Parameters/1(P) -> PID Controller/2
  TR/1 -> PID Controller/6
  Error/1 -> PID Controller/1
  PID Controller/1 -> Out1/1

== system Controller_without_ref/decController/vel z ==
  Error : Inport
  TR : Inport  Port=2
  PID Controller : simulink/Continuous/PID Controller  Controller=PID  TimeDomain=Discrete-time  SampleTime=-1  IntegratorMethod=Forward Euler  FilterMethod=Forward Euler  Form=Parallel  UseFilter=on  ControllerParametersSource=external  P=1  I=1  D=0  N=100  InitialConditionSource=internal  InitialConditionForIntegrator=0  InitialConditionForFilter=0  ExternalReset=none  LimitOutput=on  UpperSaturationLimit=1  LowerSaturationLimit=-1  LinearizeAsGain=on  AntiWindupMode=clamping  Kb=1  TrackingMode=on  Kt=1  SaturateOnIntegerOverflow=on  PParamMin=[]  PParamMax=[]  IParamMin=[]  IParamMax=[]  DParamMin=[]  DParamMax=[]  NParamMin=[]  NParamMax=[]  KbParamMin=[]  KbParamMax=[]  KtParamMin=[]  KtParamMax=[]  POutMin=[]  POutMax=[]  IOutMin=[]  IOutMax=[]  DOutMin=[]  DOutMax=[]  NOutMin=[]  NOutMax=[]  KbOutMin=[]  KbOutMax=[]  KtOutMin=[]  KtOutMax=[]  IntegratorOutMin=[]  IntegratorOutMax=[]  FilterOutMin=[]  FilterOutMax=[]  SumOutMin=[]  SumOutMax=[]  SumI1OutMin=[]  SumI1OutMax=[]  SumI2OutMin=[]  SumI2OutMax=[]  SumI3OutMin=[]  SumI3OutMax=[]  SumDOutMin=[]  SumDOutMax=[]  SaturationOutMin=[]  SaturationOutMax=[]  IntegratorContinuousStateAttributes=''  IntegratorStateMustResolveToSignalObject=off  IntegratorRTWStateStorageClass=Auto  FilterContinuousStateAttributes=''  FilterStateMustResolveToSignalObject=off  FilterRTWStateStorageClass=Auto  DifferentiatorICPrevScaledInput=0  DifferentiatorOutMin=[]  DifferentiatorOutMax=[]
  Retrive PID-Parameters : Subsystem
  Out1 : Outport
  wires:
  Retrive PID-Parameters/3(D) -> PID Controller/4
  Retrive PID-Parameters/2(I) -> PID Controller/3
  Retrive PID-Parameters/4(N) -> PID Controller/5
  Retrive PID-Parameters/1(P) -> PID Controller/2
  TR/1 -> PID Controller/6
  Error/1 -> PID Controller/1
  PID Controller/1 -> Out1/1

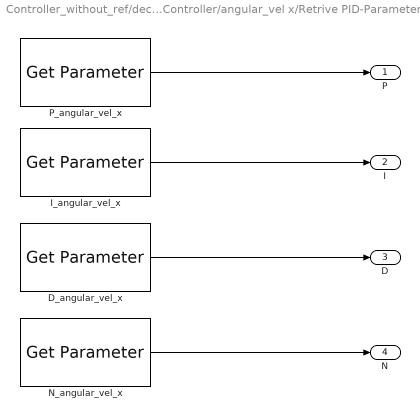
== system Controller_without_ref/decController/angular_vel x/Retrive PID-Parameters ==
  D_angular_vel_x : robotlib/Get Parameter  SourceLibraryInfo=This block requires Robotics System Toolbox  ParameterSource=Select from ROS network  ParameterName=/matlab_controller/D_angular_vel_x  ParameterType=double  ParameterInitialValue=0  SampleTime=-1  ShowErrorCodeOutput=off  ModelName=Controller_without_ref  BlockId=ParamGet_Controller_without_ref_505
  I_angular_vel_x : robotlib/Get Parameter  SourceLibraryInfo=This block requires Robotics System Toolbox  ParameterSource=Select from ROS network  ParameterName=/matlab_controller/I_angular_vel_x  ParameterType=double  ParameterInitialValue=0  SampleTime=-1  ShowErrorCodeOutput=off  ModelName=Controller_without_ref  BlockId=ParamGet_Controller_without_ref_506
  "N_angular_vel_x " : robotlib/Get Parameter  SourceLibraryInfo=This block requires Robotics System Toolbox  ParameterSource=Specify your own  ParameterName=/matlab_controller/N_angular_vel_x  ParameterType=double  ParameterInitialValue=0  SampleTime=-1  ShowErrorCodeOutput=off  ModelName=Controller_without_ref  BlockId=ParamGet_Controller_without_ref_507
  P_angular_vel_x : robotlib/Get Parameter  SourceLibraryInfo=This block requires Robotics System Toolbox  ParameterSource=Select from ROS network  ParameterName=/matlab_controller/P_angular_vel_x  ParameterType=double  ParameterInitialValue=0  SampleTime=-1  ShowErrorCodeOutput=off  ModelName=Controller_without_ref  BlockId=ParamGet_Controller_without_ref_508
  P : Outport
  I : Outport  Port=2
  D : Outport  Port=3
  N : Outport  Port=4
  wires:
  "N_angular_vel_x "/1 -> N/1
  D_angular_vel_x/1 -> D/1
  I_angular_vel_x/1 -> I/1
  P_angular_vel_x/1 -> P/1

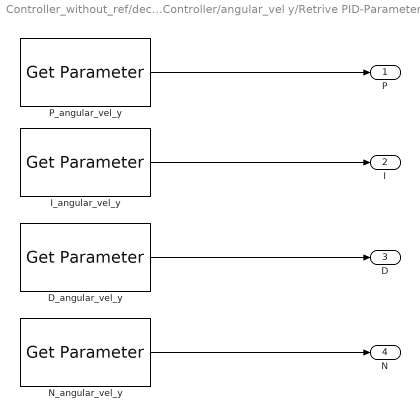
== system Controller_without_ref/decController/angular_vel y/Retrive PID-Parameters ==
  D_angular_vel_y : robotlib/Get Parameter  SourceLibraryInfo=This block requires Robotics System Toolbox  ParameterSource=Specify your own  ParameterName=/matlab_controller/D_angular_vel_y  ParameterType=double  ParameterInitialValue=0  SampleTime=-1  ShowErrorCodeOutput=off  ModelName=Controller_without_ref  BlockId=ParamGet_Controller_without_ref_519
  I_angular_vel_y : robotlib/Get Parameter  SourceLibraryInfo=This block requires Robotics System Toolbox  ParameterSource=Specify your own  ParameterName=/matlab_controller/I_angular_vel_y  ParameterType=double  ParameterInitialValue=0  SampleTime=-1  ShowErrorCodeOutput=off  ModelName=Controller_without_ref  BlockId=ParamGet_Controller_without_ref_520
  "N_angular_vel_y " : robotlib/Get Parameter  SourceLibraryInfo=This block requires Robotics System Toolbox  ParameterSource=Specify your own  ParameterName=/matlab_controller/N_angular_vel_y  ParameterType=double  ParameterInitialValue=0  SampleTime=-1  ShowErrorCodeOutput=off  ModelName=Controller_without_ref  BlockId=ParamGet_Controller_without_ref_521
  P_angular_vel_y : robotlib/Get Parameter  SourceLibraryInfo=This block requires Robotics System Toolbox  ParameterSource=Specify your own  ParameterName=/matlab_controller/P_angular_vel_y  ParameterType=double  ParameterInitialValue=0  SampleTime=-1  ShowErrorCodeOutput=off  ModelName=Controller_without_ref  BlockId=ParamGet_Controller_without_ref_522
  P : Outport
  I : Outport  Port=2
  D : Outport  Port=3
  N : Outport  Port=4
  wires:
  "N_angular_vel_y "/1 -> N/1
  D_angular_vel_y/1 -> D/1
  I_angular_vel_y/1 -> I/1
  P_angular_vel_y/1 -> P/1

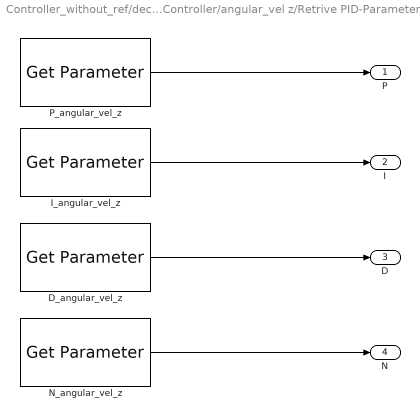
== system Controller_without_ref/decController/angular_vel z/Retrive PID-Parameters ==
  D_angular_vel_z : robotlib/Get Parameter  SourceLibraryInfo=This block requires Robotics System Toolbox  ParameterSource=Specify your own  ParameterName=/matlab_controller/D_angular_vel_z  ParameterType=double  ParameterInitialValue=0  SampleTime=-1  ShowErrorCodeOutput=off  ModelName=Controller_without_ref  BlockId=ParamGet_Controller_without_ref_533
  I_angular_vel_z : robotlib/Get Parameter  SourceLibraryInfo=This block requires Robotics System Toolbox  ParameterSource=Specify your own  ParameterName=/matlab_controller/I_angular_vel_z  ParameterType=double  ParameterInitialValue=0  SampleTime=-1  ShowErrorCodeOutput=off  ModelName=Controller_without_ref  BlockId=ParamGet_Controller_without_ref_534
  "N_angular_vel_z " : robotlib/Get Parameter  SourceLibraryInfo=This block requires Robotics System Toolbox  ParameterSource=Specify your own  ParameterName=/matlab_controller/N_angular_vel_z  ParameterType=double  ParameterInitialValue=0  SampleTime=-1  ShowErrorCodeOutput=off  ModelName=Controller_without_ref  BlockId=ParamGet_Controller_without_ref_535
  P_angular_vel_z : robotlib/Get Parameter  SourceLibraryInfo=This block requires Robotics System Toolbox  ParameterSource=Specify your own  ParameterName=/matlab_controller/P_angular_vel_z  ParameterType=double  ParameterInitialValue=0  SampleTime=-1  ShowErrorCodeOutput=off  ModelName=Controller_without_ref  BlockId=ParamGet_Controller_without_ref_536
  P : Outport
  I : Outport  Port=2
  D : Outport  Port=3
  N : Outport  Port=4
  wires:
  "N_angular_vel_z "/1 -> N/1
  D_angular_vel_z/1 -> D/1
  I_angular_vel_z/1 -> I/1
  P_angular_vel_z/1 -> P/1

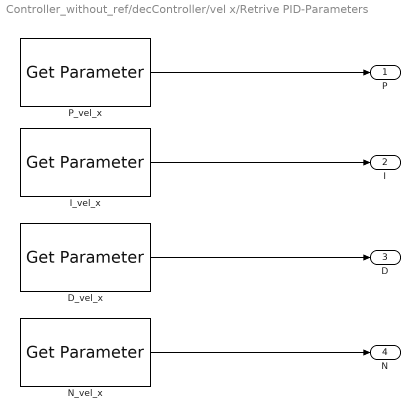
== system Controller_without_ref/decController/vel x/Retrive PID-Parameters ==
  D_vel_x : robotlib/Get Parameter  SourceLibraryInfo=This block requires Robotics System Toolbox  ParameterSource=Specify your own  ParameterName=/matlab_controller/D_vel_x  ParameterType=double  ParameterInitialValue=0  SampleTime=-1  ShowErrorCodeOutput=off  ModelName=Controller_without_ref  BlockId=ParamGet_Controller_without_ref_547
  I_vel_x : robotlib/Get Parameter  SourceLibraryInfo=This block requires Robotics System Toolbox  ParameterSource=Specify your own  ParameterName=/matlab_controller/I_vel_x  ParameterType=double  ParameterInitialValue=0  SampleTime=-1  ShowErrorCodeOutput=off  ModelName=Controller_without_ref  BlockId=ParamGet_Controller_without_ref_548
  "N_vel_x " : robotlib/Get Parameter  SourceLibraryInfo=This block requires Robotics System Toolbox  ParameterSource=Specify your own  ParameterName=/matlab_controller/N_vel_x  ParameterType=double  ParameterInitialValue=0  SampleTime=-1  ShowErrorCodeOutput=off  ModelName=Controller_without_ref  BlockId=ParamGet_Controller_without_ref_549
  P_vel_x : robotlib/Get Parameter  SourceLibraryInfo=This block requires Robotics System Toolbox  ParameterSource=Specify your own  ParameterName=/matlab_controller/P_vel_x  ParameterType=double  ParameterInitialValue=0  SampleTime=-1  ShowErrorCodeOutput=off  ModelName=Controller_without_ref  BlockId=ParamGet_Controller_without_ref_550
  P : Outport
  I : Outport  Port=2
  D : Outport  Port=3
  N : Outport  Port=4
  wires:
  "N_vel_x "/1 -> N/1
  D_vel_x/1 -> D/1
  I_vel_x/1 -> I/1
  P_vel_x/1 -> P/1

== system Controller_without_ref/decController/vel y/Retrive PID-Parameters ==
  D_vel_y : robotlib/Get Parameter  SourceLibraryInfo=This block requires Robotics System Toolbox  ParameterSource=Specify your own  ParameterName=/matlab_controller/D_vel_y  ParameterType=double  ParameterInitialValue=0  SampleTime=-1  ShowErrorCodeOutput=off  ModelName=Controller_without_ref  BlockId=ParamGet_Controller_without_ref_561
  I_vel_y : robotlib/Get Parameter  SourceLibraryInfo=This block requires Robotics System Toolbox  ParameterSource=Specify your own  ParameterName=/matlab_controller/I_vel_y  ParameterType=double  ParameterInitialValue=0  SampleTime=-1  ShowErrorCodeOutput=off  ModelName=Controller_without_ref  BlockId=ParamGet_Controller_without_ref_562
  "N_vel_y " : robotlib/Get Parameter  SourceLibraryInfo=This block requires Robotics System Toolbox  ParameterSource=Specify your own  ParameterName=/matlab_controller/N_vel_y  ParameterType=double  ParameterInitialValue=0  SampleTime=-1  ShowErrorCodeOutput=off  ModelName=Controller_without_ref  BlockId=ParamGet_Controller_without_ref_563
  P_vel_y : robotlib/Get Parameter  SourceLibraryInfo=This block requires Robotics System Toolbox  ParameterSource=Specify your own  ParameterName=/matlab_controller/P_vel_y  ParameterType=double  ParameterInitialValue=0  SampleTime=-1  ShowErrorCodeOutput=off  ModelName=Controller_without_ref  BlockId=ParamGet_Controller_without_ref_564
  P : Outport
  I : Outport  Port=2
  D : Outport  Port=3
  N : Outport  Port=4
  wires:
  "N_vel_y "/1 -> N/1
  D_vel_y/1 -> D/1
  I_vel_y/1 -> I/1
  P_vel_y/1 -> P/1

== system Controller_without_ref/decController/vel z/Retrive PID-Parameters ==
  D_vel_z : robotlib/Get Parameter  SourceLibraryInfo=This block requires Robotics System Toolbox  ParameterSource=Specify your own  ParameterName=/matlab_controller/D_vel_z  ParameterType=double  ParameterInitialValue=0  SampleTime=-1  ShowErrorCodeOutput=off  ModelName=Controller_without_ref  BlockId=ParamGet_Controller_without_ref_575
  I_vel_z : robotlib/Get Parameter  SourceLibraryInfo=This block requires Robotics System Toolbox  ParameterSource=Specify your own  ParameterName=/matlab_controller/I_vel_z  ParameterType=double  ParameterInitialValue=0  SampleTime=-1  ShowErrorCodeOutput=off  ModelName=Controller_without_ref  BlockId=ParamGet_Controller_without_ref_576
  "N_vel_z " : robotlib/Get Parameter  SourceLibraryInfo=This block requires Robotics System Toolbox  ParameterSource=Specify your own  ParameterName=/matlab_controller/N_vel_z  ParameterType=double  ParameterInitialValue=0  SampleTime=-1  ShowErrorCodeOutput=off  ModelName=Controller_without_ref  BlockId=ParamGet_Controller_without_ref_577
  P_vel_z : robotlib/Get Parameter  SourceLibraryInfo=This block requires Robotics System Toolbox  ParameterSource=Specify your own  ParameterName=/matlab_controller/P_vel_z  ParameterType=double  ParameterInitialValue=0  SampleTime=-1  ShowErrorCodeOutput=off  ModelName=Controller_without_ref  BlockId=ParamGet_Controller_without_ref_578
  P : Outport
  I : Outport  Port=2
  D : Outport  Port=3
  N : Outport  Port=4
  wires:
  "N_vel_z "/1 -> N/1
  D_vel_z/1 -> D/1
  I_vel_z/1 -> I/1
  P_vel_z/1 -> P/1

== matlab function Controller_without_ref/mavros_data/Conversion ==
  data: yaw output; x input; y input; z input; w input; pitch output; roll output
function [yaw,pitch,roll]  = quat2eul(x,y,z,w)
%#codegen

% Convert the quaternion to a yaw angle (zyx euler angle)
eul = quat2eul([w,x,y,z]);
yaw = 180/pi*(-eul(1));
pitch = 180/pi*(-eul(2));
roll = 180/pi*(eul(3));

end

== matlab function Controller_without_ref/Decouple/MATLAB Function ==
  data: angular_x input; thruster1 output; angular_y input; angular_z input; vel_x input; vel_y input; vel_z input; front_strafe_decouple input; front_forward_decouple input; front_pitch_bias input; front_vertical_bias input; buoyancy_control input; thruster2 output; thruster3 output; thruster4 output; thruster5 output; thruster6 output
function [thruster1,thruster2,thruster3,thruster4,thruster5,thruster6] =...
    basicdecouple(angular_x,angular_y,angular_z,vel_x,vel_y,vel_z,...
    front_strafe_decouple,front_forward_decouple,front_pitch_bias,...
    front_vertical_bias,buoyancy_control)

% Vertical Left thruster (VL)
thruster1 =...
    angular_x...
    -front_forward_decouple*vel_x...
    -front_strafe_decouple*vel_y...
    -front_pitch_bias*angular_y...
    +front_vertical_bias*vel_z...
    +buoyancy_control; 


% Vertical Back thruster (VB)
thruster2 =...
    front_forward_decouple * vel_x...
    +angular_y...
    +vel_z...
    +buoyancy_control; 


thruster3 =...
    -angular_x...
    -front_forward_decouple * vel_x+...
    front_strafe_decouple*vel_y...
    -front_pitch_bias*angular_y...
    +front_vertical_bias * vel_z...
    +buoyancy_control;

 %Forward Left (FL)
thruster4 =...
    -angular_z...
    + vel_x;
thruster5 = vel_y; % LATeral (LAT)

% Forward Right (FR)
thruster6 =...
    angular_z...
    + vel_x;

end

== matlab function Controller_without_ref/mavros_data/removeGravity ==
  data: w input; x input; y input; z input; x_acc input; y_acc input; z_acc input; x_accnew output; y_accnew output; z_accnew output
function [x_accnew,y_accnew,z_accnew]  = removeGravity(w,x,y,z,x_acc,y_acc,z_acc)
%#codegen

rotmatrix = [2*w^2+2*x^2-1, 2*x*y-2*w*z, 2*x*z+2*w*y; 
    2*x*y+2*w*z, 2*w^2+2*y^2-1, 2*x*z-2*w*x;
    2*x*z-2*w*y, 2*y*z+2*w*x, 2*w^2+2*z^2-1];

g = [0;0;-9.79];
% Gravity projected in the body fixed frame
acc = inv(rotmatrix)*g;

% Removed gravity from the acceleration
x_accnew = x_acc+acc(1);
y_accnew = y_acc+acc(2);
z_accnew = z_acc+acc(3);
end

== matlab function Controller_without_ref/toPWM/Calc pwm signal ==
  data: controlsignal input; pwm output
function pwm = calcPWM(controlsignal)
 % thruster values should be between 1100 and 1900 microseconds (us)
 % values less than 1500 us are backwards; values more than are forwards

pwm=(controlsignal + 1) * 400 + 1100;

end
